simulink model "Robot_Control_v01"  (Simulink 8.4)
settings: Solver=ode45  StartTime=0.0  StopTime=10.0  RelTol=1e-3
values from neighbouring files (symbols this model uses):
  q0 = [-32;-5;0]    [main_v01.m]
settings Model: Creator=farbod  LastModifiedBy=sd0016
settings SFSimCC: SimParseCustomCode=off

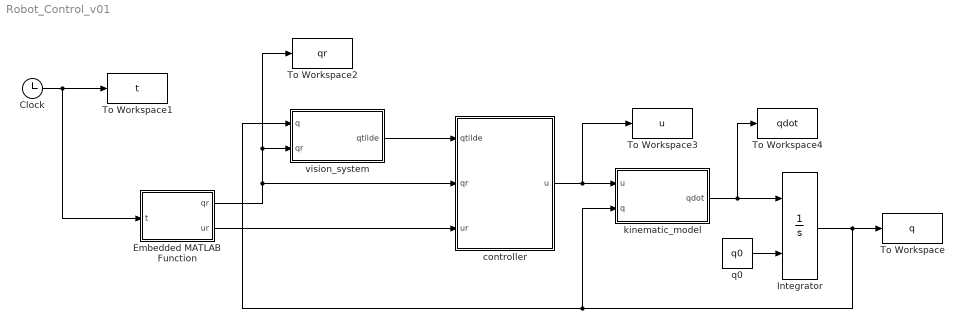
== system Robot_Control_v01 ==
  Clock : Clock
  Embedded MATLAB Function : MATLAB Function  TreatAsAtomicUnit=on
  Integrator : Integrator  InitialConditionSource=external
  To Workspace : ToWorkspace  VariableName=q  SampleTime=-1
  To Workspace1 : ToWorkspace  VariableName=t  SampleTime=-1
  To Workspace2 : ToWorkspace  VariableName=qr  SampleTime=-1
  To Workspace3 : ToWorkspace  VariableName=u  SampleTime=-1
  To Workspace4 : ToWorkspace  VariableName=qdot  SampleTime=-1
  controller : MATLAB Function  TreatAsAtomicUnit=on
  kinematic_model : MATLAB Function  TreatAsAtomicUnit=on
  q0 : Constant  Value=q0
  vision_system : MATLAB Function  TreatAsAtomicUnit=on
  wires:
  kinematic_model/1(qdot) -> Integrator/1, To Workspace4/1
  q0/1 -> Integrator/2
  Integrator/1 -> To Workspace/1, kinematic_model/2(q), vision_system/1(q)
  controller/1(u) -> kinematic_model/1(u), To Workspace3/1
  Clock/1 -> To Workspace1/1, Embedded MATLAB Function/1(t)
  vision_system/1(qtilde) -> controller/1(qtilde)
  Embedded MATLAB Function/1(qr) -> controller/2(qr), vision_system/2(qr), To Workspace2/1
  Embedded MATLAB Function/2(ur) -> controller/3(ur)

== matlab function controller ==
  data: u output double; qtilde input double; qr input double; ur input double
function u = controller(qtilde,qr,ur)
% the controller
% u = [v omega]^T
% qtilde: posture error
% qr    : reference (desired) posture

%%----------Input Parametleri Duzenleniyor---------------------------------

u = zeros(2,1);

% for now
vr     = ur(1,1);
omegar = ur(2,1);

% According to the vision system: qtilde = q - qr, so
q = qtilde + qr;

xr     = qr(1,1);
yr     = qr(2,1);
thetar = qr(3,1);

x     = q(1,1);
y     = q(2,1);
theta = q(3,1);

s = sin(theta);
c = cos(theta);

%% -------------------------Error Hesaplaniyor----------------------------
% Burada temelde 3 tane olan hata parametreleri 4 e cikariliyor. 
% theta parametresi es ve ec olarak iki ayri hata parametresine cevriliyor

% Eq.(4), third element!
etheta = thetar-theta;

% Local errors from Eq.(10)
ex = c*(xr - x) + s*(yr - y);
ey = -s*(xr - x) + c*(yr - y);

es = sin(thetar-theta);
ecos = cos(thetar-theta);

ec = ecos -1;

%--------------------------------------------------------------------------
%% - u ya ulasabilmek icin ihtiyacimiz olanlar
% vb,omegab,vr,omegar: ilk ikisi hesaplaniyor son ikisi ur'den geliyor.
% k,kx,ks,a,n paper temel alinarak secilmis secilmis

% according to the paper
k = 1; % k > 0
kx = 1; % kx(t) > 0
ks = 1; % ks(t) > 0
a = 3; % a > 2
n = 0; % n = -2, -1, 0, 1 or 2

% Eq.(18)
vb = kx*ex;
omegab = k*vr*ey*(1+ec/a)^2+ks*es*((1+ec/a)^2)^n;

u = [vr*cos(etheta)+vb; omegar+omegab]; % Eq.(6)

%buradaki u degeri controllerdan cikan ve sisteme giris olarak verilen u

== matlab function kinematic_model ==
  data: u input double; q input double; qdot output double
function qdot = kinematic(u,q)
% Kinematic Model

% q = [x y theta]^T
% qdot = [xdot ydot thetadot]^T
% u = [v omega]^T

qdot = zeros(3,1);

theta = q(3);

qdot = [cos(theta),0;sin(theta),0;0,1]*u; % Eq.(2)

== matlab function vision_system ==
  data: q input double; qtilde output double; qr input double
function qtilde  = error(q,qr)
%#codegen

    %Camera System simulation
    %Takes the position of the robot in I space and returns left and right
    %target pixel values.
    %In real application L_p and R_p will come from physical camera system.

    p1x = 0;
    p1y = 0;
    p1z = 0;

%     P = zeros(4,4);
%     P(:,1) = [p1x, p1y, p1z, 1];
%     P(:,2) = [p1x, p1y+8, p1z, 1];
%     P(:,3) = [p1x+8, p1y+4, p1z+3, 1];
%     P(:,4) = [p1x, p1y+4, p1z+8, 1];
    P = zeros(4,4);
    P(1,:) = random(-5,5,4);
    P(2,:) = random(-5,5,4);
    P(3,:) = random(-5,5,4);
    P(4,:) = ones(1,4);

    %Define Intrinsic Params
    f = 800;
    pp = [320 240];
    
    nl = 10;
    noise = random(-nl,nl,size(P,2));
    
    %Define Robot
    robotPose = newPose(q(1),q(2),0,0,0,q(3));
    robotPoseDes = newPose(qr(1),qr(2),0,0,0,qr(3));

    world2robotDes = inv(transformationMatrix(robotPoseDes));

    [L_p, R_p, S_PDes, robot] = setupPointsAndPixels(robotPose,robotPoseDes,P,800,[320 240]);

    %Add noise to the pixels

%     L_p = [L_p(1,:)+noise'; L_p(2,:)+noise'];    
%     R_p = [R_p(1,:)+noise'; R_p(2,:)+noise']; 

    %Pose estimation
    param = mirage(robot, S_PDes, L_p, R_p)';

    sol = eye(4,4); sol(1:3,:) = reshape(param,3,4);

    world2robot = sol*world2robotDes;

    [~, ~, psi] = get3DRotationAngles((world2robot(1:3,1:3)));

    qtilde = zeros(3,1);
    qtilde(1) = -world2robot(1,4)   - qr(1);
    qtilde(2) = -world2robot(2,4)   - qr(2);
    qtilde(3) = -psi                - qr(3);
end

function [L_p, R_p, S_PDes, robot] = setupPointsAndPixels(pose,robotPoseDes,P,f,pp)
    % Setup for PROPOSED METHOD

    %define camera Poses with respect to the robot
    leftCamPose = newPose(2,1,1,0,0,0);
    rightCamPose = newPose(2,-1,1,0,0,0);

    %define cameras 
    leftCamera = newCamera(leftCamPose,f,f,pp(2),pp(1),0,0);
    rightCamera = newCamera(rightCamPose,f,f,pp(2),pp(1),0,0);

    %Define Robot
    robot = newRobot(pose, leftCamera, rightCamera);

    world2robotDes = inv(transformationMatrix(robotPoseDes));
    S_PDes = world2robotDes * P;

    [L_p, R_p] = simulateRealRobot(P,robot);
end

== matlab function Embedded MATLAB Function ==
  data: t input double; qr output double; ur output double
function [qr,ur] = desired(t)
%#eml

% qr = [xr yr thetar]^T (reference trajectory)
% ur = [vr omegar]^T (reference control input that generates the reference trajetory in ideal conditions)

A = 1;
xL = 10;
vx = 1;

% % 
% % desired x and y 
% xr = vx*t;
% yr = A*sin(2*pi*xr/xL);
% 
% % desired x and y derivatives
% xrdot = vx;
% yrdot = A*(2*pi/xL)*cos(2*pi*xr/xL);
% 
% % desired theta
% thetar = atan2(yrdot,xrdot);
% 
% % desired second derivatives
% xrddot = 0;
% yrddot = -A*(2*pi/xL)^2*sin(2*pi*xr/xL);
% 
% % desired theta derivative
% thetardot = (yrddot - xrddot*tan(thetar))/(xrdot*(1+tan(thetar)^2));
% 
% 
% vr     = sqrt(xrdot^2+yrdot^2);
% omegar = thetardot;

%--------------------------------------------
% 
xr = vx*t - 30;
yr = A*sin(2*pi*xr/xL) + 2;

% desired x and y derivatives
xrdot = vx;
yrdot = A*(2*pi/xL)*cos(2*pi*xr/xL);

% desired theta
thetar = atan2(yrdot,xrdot);

% desired second derivatives
xrddot = 0;
yrddot = -A*(2*pi/xL)^2*sin(2*pi*xr/xL);

% desired theta derivative
thetardot = (yrddot - xrddot*tan(thetar))/(xrdot*(1+tan(thetar)^2));

vr     = sqrt(xrdot^2+yrdot^2);
omegar = thetardot;

%--------------------------------------------
% yr = vx*t - 30;
% xr = A*sin(2*pi*yr/xL) + 2;
% 
% yrdot = vx;
% xrdot = A*(2*pi/xL)*cos(2*pi*xr/xL);
% 
% desired theta
% thetar = atan2(yrdot,xrdot);
% thetardot = 0;
% 
% vr     = sqrt(xrdot^2+yrdot^2);
% omegar = thetardot;

%--------------------------------------------
% xr = vx*t - 30;
% yr = 5;
% 
% xrdot = vx;
% yrdot = 0;
% 
% thetar = 0;
% thetardot = 0;
% 
% vr     = sqrt(xrdot^2+yrdot^2);
% omegar = thetardot;

qr = [xr;yr;thetar];
ur = [vr;omegar];
